simulink model "Simulink_AM_Mod_Demod"  (R2021a)
settings: Solver=VariableStepAuto  StartTime=0.0  StopTime=10.0  RelTol=1e-3
libraries: dspfdesign x1
settings Model: NumberOfSteps=5  Creator=visha  LastModifiedBy=visha

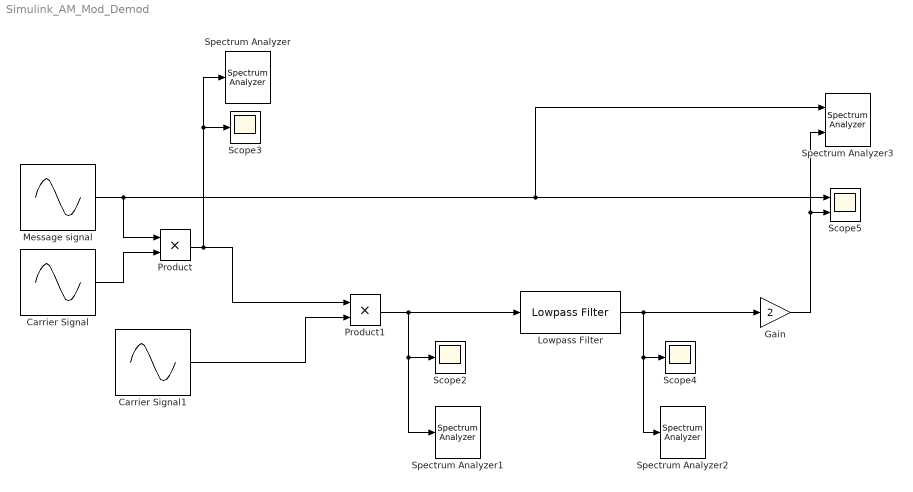
== system Simulink_AM_Mod_Demod ==
  Carrier Signal : Sin  Frequency=1000*2*pi  Phase=pi/2  SampleTime=1/2^14
  Carrier Signal1 : Sin  Frequency=1000*2*pi  Phase=pi/2  SampleTime=1/2^14
  Gain : Gain  Gain=2
  Lowpass Filter : dspfdesign/Lowpass Filter  FilterType=FIR  DesignForMinimumOrder=off  FilterOrder=50  PassbandFrequency=0.1e3  StopbandFrequency=1e3  PassbandRipple=0.1  StopbandAttenuation=80  InheritSampleRate=off  SampleRate=44100  SimulateUsing=Interpreted execution  roundingMode=Floor  coeffsDataTypeStr=fixdt(1,16)
  Message signal : Sin  Frequency=100*2*pi  SampleTime=1/2^14
  Product : Product
  Product1 : Product
  Scope2 : Scope
  Scope3 : Scope
  Scope4 : Scope
  Scope5 : Scope  NumInputPorts=2
  Spectrum Analyzer : SpectrumAnalyzer
  Spectrum Analyzer1 : SpectrumAnalyzer
  Spectrum Analyzer2 : SpectrumAnalyzer
  Spectrum Analyzer3 : SpectrumAnalyzer  NumInputPorts=2
  wires:
  Message signal/1 -> Spectrum Analyzer3/1, Scope5/1, Product/1
  Carrier Signal/1 -> Product/2
  Product/1 -> Product1/1, Spectrum Analyzer/1, Scope3/1
  Carrier Signal1/1 -> Product1/2
  Product1/1 -> Lowpass Filter/1, Spectrum Analyzer1/1, Scope2/1
  Lowpass Filter/1 -> Gain/1, Spectrum Analyzer2/1, Scope4/1
  Gain/1 -> Spectrum Analyzer3/2, Scope5/2
